simulink model "model_sim"  (R2022a)
settings: Solver=VariableStepAuto  StartTime=0.0  StopTime=40.0  RelTol=1e-3
values from neighbouring files (symbols this model uses):
  beta = params(1)    [model.m]
  g = 9.8105    [model.m]    (also in weryfikacja.m)
  I = 0.029572173408016    (= 0.029572173408)    [model.m]    (also in weryfikacja.m)
  K = params(3)    [model.m]
  K_lqr = lqr(A,B,Q,R)    [weryfikacja.m]
  mu1 = params(11:end)    [model.m]
  p1 = params(5:10)    [model.m]    (also in weryfikacja.m)
  tau = params(4)    [model.m]
  U = params(2)    [model.m]
  xep = [deg2rad(-2*21.37) 0 2000]    [weryfikacja.m]
settings Model: Creator=turgo  LastModifiedBy=turgo

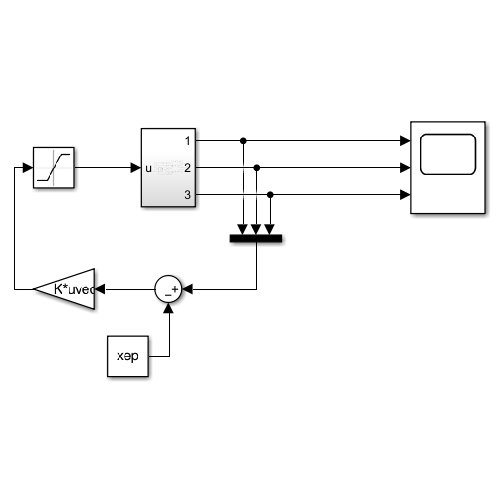
[thumbnail: Simulink's stored preview of the top-level diagram]
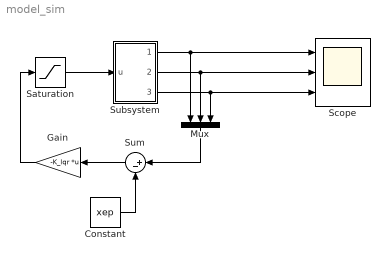
== system model_sim ==
  Constant : Constant  Value=xep  VectorParams1D=off
  Gain : Gain  Gain=-K_lqr  Multiplication=Matrix(K*u) (u vector)
  Mux : Mux  Inputs=3
  Saturation : Saturate  UpperLimit=0.8  LowerLimit=-0.8
  Scope : Scope  NumInputPorts=3
  Subsystem : Subsystem
  Sum : Sum  Inputs=|+-
  wires:
  Subsystem/1(Out1) -> Scope/1, Mux/1
  Subsystem/2(Out2) -> Mux/2, Scope/2
  Subsystem/3(Out3) -> Mux/3, Scope/3
  Constant/1 -> Sum/2
  Sum/1 -> Gain/1
  Mux/1 -> Sum/1
  Saturation/1 -> Subsystem/1(u)
  Gain/1 -> Saturation/1

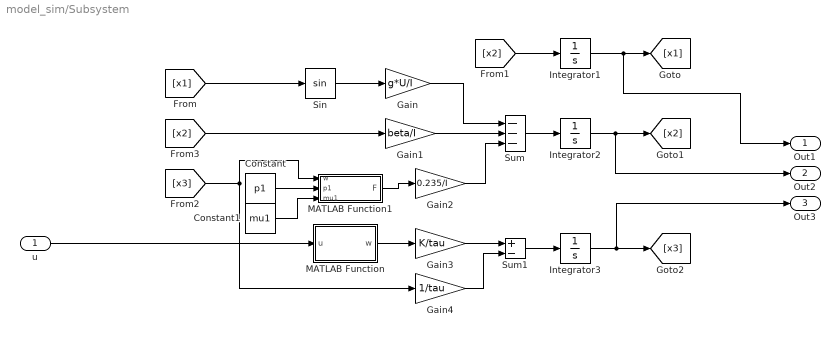
== system model_sim/Subsystem ==
  u : Inport
  Constant : Constant  Value=p1  VectorParams1D=off
  Constant1 : Constant  Value=mu1
  Gain : Gain  Gain=g*U/I
  Gain1 : Gain  Gain=beta/I
  Gain2 : Gain  Gain=0.235/I
  Gain3 : Gain  Gain=K/tau
  Gain4 : Gain  Gain=1/tau
  Integrator1 : Integrator
  Integrator2 : Integrator
  Integrator3 : Integrator
  MATLAB Function : MATLAB Function  TreatAsAtomicUnit=on
  MATLAB Function1 : MATLAB Function  TreatAsAtomicUnit=on
  Sin : Trigonometry
  Sum : Sum  Inputs=---
  Sum1 : Sum  Inputs=+-
  Out1 : Outport
  Out2 : Outport  Port=2
  Out3 : Outport  Port=3
  wires:
  [x1] -> Sin/1
  [x3] -> Gain4/1, MATLAB Function1/1(w)
  Integrator1/1 -> Out1/1, [x1]
  Sum/1 -> Integrator2/1
  Sum1/1 -> Integrator3/1
  Sin/1 -> Gain/1
  MATLAB Function1/1(F) -> Gain2/1
  Gain/1 -> Sum/1
  Gain2/1 -> Sum/3
  Constant1/1 -> MATLAB Function1/3(mu1)
  Gain4/1 -> Sum1/2
  Gain3/1 -> Sum1/1
  [x2] -> Gain1/1
  [x2] -> Integrator1/1
  MATLAB Function/1(w) -> Gain3/1
  Constant/1 -> MATLAB Function1/2(p1)
  Integrator3/1 -> Out3/1, [x3]
  Gain1/1 -> Sum/2
  Integrator2/1 -> Out2/1, [x2]
  u/1 -> MATLAB Function/1(u)

== matlab function model_sim/Subsystem/MATLAB Function1 ==
  data: w input; F output; p1 input; mu1 input
function F  = model_sila_ciagu(w, p1, mu1)
    F = polyval(p1, w,[],mu1);
    F = min(max(F,-0.65),0.8);
end

== matlab function model_sim/Subsystem/MATLAB Function ==
  data: u input; w output
function w  = model_sterowanie(u)
    p2 = [2.056467854285133e+02,-5.208575031241387,-1.043284835310092e+03,43.401332957404660,3.454345824430912e+03,1.802723922744937];
    mu2 = [0;0.636602825861413];
    w = polyval(p2, u, [], mu2);
end
